simulink subsystem "Read_RC"  (R2025a)
settings: Solver=VariableStepAuto  StartTime=0.0  StopTime=10.0  RelTol=1e-3
libraries: px4uORBlib x1
settings Model: Creator=gurt1  LastModifiedBy=17036
settings RTWCC: GPUComputeCapability=3.5

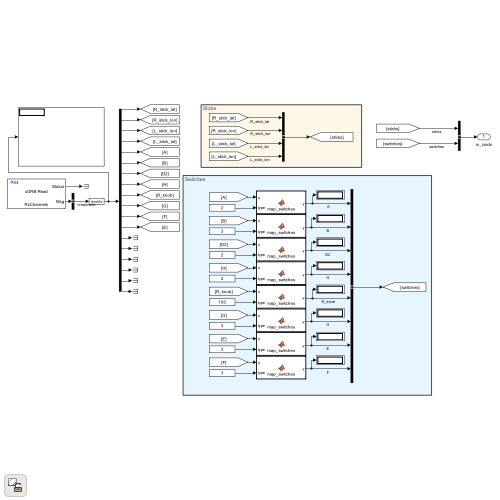
[thumbnail: Simulink's stored preview of the top-level diagram]
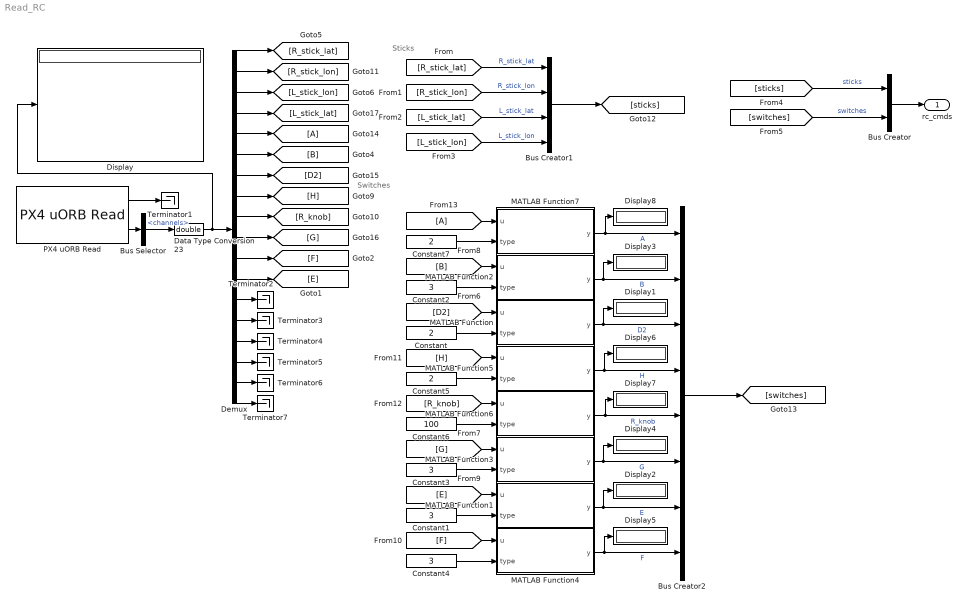
== system Read_RC ==
  note: Switches
  note: Sticks
  Bus Creator : BusCreator  Inputs=2
  Bus Creator1 : BusCreator  Inputs=4
  Bus Creator2 : BusCreator  Inputs=8
  Bus Selector : BusSelector  OutputSignals=channels
  Constant : Constant  Value=2
  Constant{1..4} (4 alike) : Constant  Value=3
  Constant5 : Constant  Value=2
  Constant6 : Constant  Value=100
  Constant7 : Constant  Value=2
  Data Type Conversion23 : DataTypeConversion  OutDataTypeStr=double  SaturateOnIntegerOverflow=off  RndMeth=Floor
  Demux : Demux  Outputs=18
  Display{,1..8} (9 alike) : Display
  From13 : From
  Goto14 : Goto
  MATLAB Function : MATLAB Function  TreatAsAtomicUnit=on
  MATLAB Function1 : MATLAB Function  TreatAsAtomicUnit=on
  MATLAB Function2 : MATLAB Function  TreatAsAtomicUnit=on
  MATLAB Function3 : MATLAB Function  TreatAsAtomicUnit=on
  MATLAB Function4 : MATLAB Function  TreatAsAtomicUnit=on
  MATLAB Function5 : MATLAB Function  TreatAsAtomicUnit=on
  MATLAB Function6 : MATLAB Function  TreatAsAtomicUnit=on
  MATLAB Function7 : MATLAB Function  TreatAsAtomicUnit=on
  PX4 uORB Read : px4uORBlib/PX4 uORB Read  uORBTopic=RcChannels  selectInstance=RcChannels  SampleTime=-1  BlockingMode=off  BlockTimeout=1e-3
  Terminator{1..7} (7 alike) : Terminator
  rc_cmds : Outport
  wires:
  Demux/1 -> [R_stick_lat]
  Demux/2 -> [R_stick_lon]
  Demux/3 -> [L_stick_lon]
  Demux/4 -> [L_stick_lat]
  Demux/5 -> Goto14/1
  Demux/6 -> [B]
  Demux/7 -> [D2]
  Demux/8 -> [H]
  Demux/9 -> [R_knob]
  Demux/10 -> [G]
  Demux/11 -> [F]
  Demux/12 -> [E]
  Demux/13 -> Terminator2/1
  Demux/17 -> Terminator6/1
  Demux/18 -> Terminator7/1
  Demux/16 -> Terminator5/1
  Demux/15 -> Terminator4/1
  Demux/14 -> Terminator3/1
  [R_stick_lat] -> Bus Creator1/1  "R_stick_lat"
  [R_stick_lon] -> Bus Creator1/2  "R_stick_lon"
  [L_stick_lat] -> Bus Creator1/3  "L_stick_lat"
  [L_stick_lon] -> Bus Creator1/4  "L_stick_lon"
  PX4 uORB Read/1 -> Terminator1/1
  PX4 uORB Read/2 -> Bus Selector/1
  Bus Selector/1 -> Data Type Conversion23/1  "<channels>"
  Data Type Conversion23/1 -> Display/1, Demux/1
  Bus Creator1/1 -> [sticks]
  Bus Creator/1 -> rc_cmds/1
  [sticks] -> Bus Creator/1  "sticks"
  [switches] -> Bus Creator/2  "switches"
  [D2] -> MATLAB Function/1(u)
  Constant/1 -> MATLAB Function/2(type)
  MATLAB Function/1(y) -> Bus Creator2/3, Display1/1  "D2"
  Constant1/1 -> MATLAB Function1/2(type)
  MATLAB Function1/1(y) -> Bus Creator2/7, Display2/1  "E"
  Constant2/1 -> MATLAB Function2/2(type)
  MATLAB Function2/1(y) -> Bus Creator2/2, Display3/1  "B"
  Constant3/1 -> MATLAB Function3/2(type)
  MATLAB Function3/1(y) -> Bus Creator2/6, Display4/1  "G"
  Constant6/1 -> MATLAB Function6/2(type)
  Constant5/1 -> MATLAB Function5/2(type)
  Constant4/1 -> MATLAB Function4/2(type)
  Constant7/1 -> MATLAB Function7/2(type)
  MATLAB Function7/1(y) -> Bus Creator2/1, Display8/1  "A"
  MATLAB Function6/1(y) -> Bus Creator2/5, Display7/1  "R_knob"
  MATLAB Function5/1(y) -> Bus Creator2/4, Display6/1  "H"
  MATLAB Function4/1(y) -> Bus Creator2/8, Display5/1  "F"
  [E] -> MATLAB Function1/1(u)
  [B] -> MATLAB Function2/1(u)
  [G] -> MATLAB Function3/1(u)
  [F] -> MATLAB Function4/1(u)
  [H] -> MATLAB Function5/1(u)
  [R_knob] -> MATLAB Function6/1(u)
  From13/1 -> MATLAB Function7/1(u)
  Bus Creator2/1 -> [switches]

== matlab function Read_RC/MATLAB Function1 ==
  data: u input; y output; type input
function y = map_switches(u,type)

y = map_switches(u,type);

== matlab function Read_RC/MATLAB Function2 ==
  data: u input; y output; type input
function y = map_switches(u,type)

y = map_switches(u,type);

== matlab function Read_RC/MATLAB Function3 ==
  data: u input; y output; type input
function y = map_switches(u,type)

y = map_switches(u,type);

== matlab function Read_RC/MATLAB Function4 ==
  data: u input; y output; type input
function y = map_switches(u,type)

y = map_switches(u,type);

== matlab function Read_RC/MATLAB Function5 ==
  data: u input; y output; type input
function y = map_switches(u,type)

y = map_switches(u,type);

== matlab function Read_RC/MATLAB Function6 ==
  data: u input; y output; type input
function y = map_switches(u,type)

y = map_switches(u,type);

== matlab function Read_RC/MATLAB Function7 ==
  data: u input; y output; type input
function y = map_switches(u,type)

y = map_switches(u,type);

== matlab function Read_RC/MATLAB Function ==
  data: u input; y output; type input
function y = map_switches(u,type)

y = map_switches(u,type);
